simulink model "AWGN_simulink"  (R2014a)
settings: Solver=ode45  StartTime=0.0  StopTime=2e-8  RelTol=1e-3
settings Model: Creator=Kushal  LastModifiedBy=Kushal
settings SolverCC: AutoInsertRateTranBlk=on  InsertRTBMode=Always

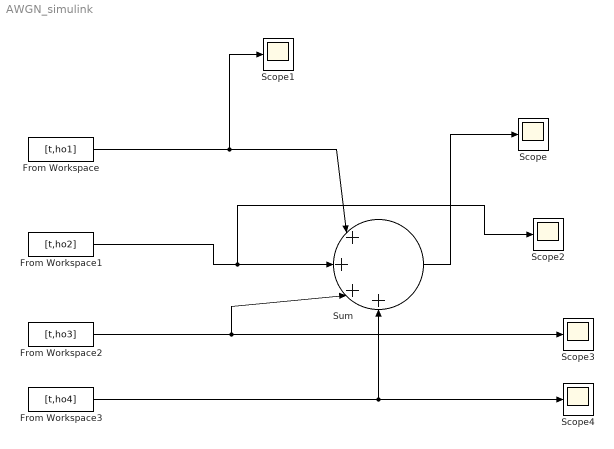
== system AWGN_simulink ==
  From Workspace : FromWorkspace  VariableName=[t,ho1]  SampleTime=0
  From Workspace1 : FromWorkspace  VariableName=[t,ho2]  SampleTime=0
  From Workspace2 : FromWorkspace  VariableName=[t,ho3]  SampleTime=0
  From Workspace3 : FromWorkspace  VariableName=[t,ho4]  SampleTime=0
  Scope{,1..4} (5 alike) : Scope
      Scope2 settings: SaveName=ScopeData2
      Scope3 settings: SaveName=ScopeData3
      Scope4 settings: SaveName=ScopeData4
  Sum : Sum  Inputs=|++++
  wires:
  From Workspace/1 -> Scope1/1, Sum/1
  From Workspace1/1 -> Scope2/1, Sum/2
  From Workspace2/1 -> Sum/3, Scope3/1
  From Workspace3/1 -> Sum/4, Scope4/1
  Sum/1 -> Scope/1
